simulink model "pcm"  (R2023b)
settings: Solver=VariableStepAuto  StartTime=0.0  StopTime=50  RelTol=1e-3
undefined symbols (not defined in the file): doppler
libraries: dspquant2 x2, dspfdesign x2, commchan3 x1
settings Model: Creator=HP  LastModifiedBy=HP

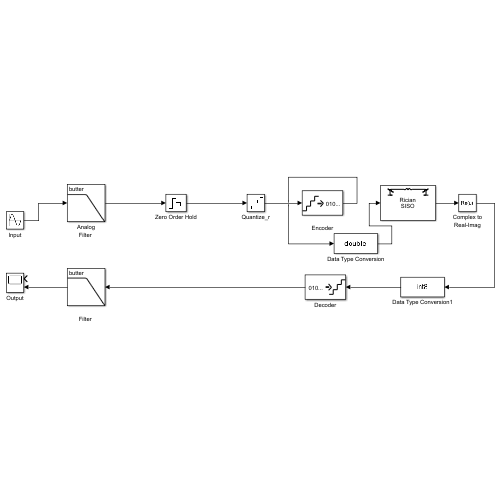
[thumbnail: Simulink's stored preview of the top-level diagram]
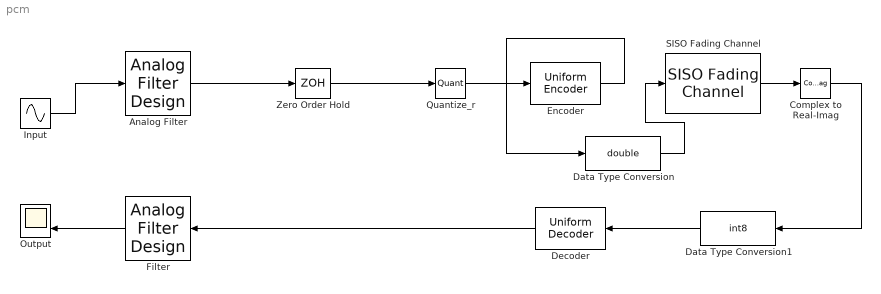
== system pcm ==
  " Encoder" : dspquant2/Uniform Encoder  peak=1  bits=3  otype=Unsigned integer
  " Filter " : dspfdesign/Analog Filter Design  method=Butterworth  filttype=Lowpass  N=8  Wlo=30  Whi=80  Rp=2  Rs=40
  "Analog Filter " : dspfdesign/Analog Filter Design  method=Butterworth  filttype=Lowpass  N=8  Wlo=30  Whi=80  Rp=2  Rs=40
  Complex to Real-Imag : ComplexToRealImag  Output=Real
  Data Type Conversion : DataTypeConversion  OutDataTypeStr=double  SaturateOnIntegerOverflow=off  RndMeth=Floor
  Data Type Conversion1 : DataTypeConversion  OutDataTypeStr=int8  SaturateOnIntegerOverflow=off  RndMeth=Floor
  Decoder : dspquant2/Uniform Decoder  peak=1  bits=8  overflowMode=Saturate  otype=Double
  Input : Sin  Amplitude=5  Frequency=5  SampleTime=0
  Output : Scope  NumInputPorts=2
  Quantize_r : Quantizer  QuantizationInterval=1
  SISO Fading Channel : commchan3/SISO Fading Channel  InheritSampleRate=on  SampleRate=1  PathDelays=0  AveragePathGains=0  NormalizePathGains=on  FadingDistribution=Rician  KFactor=3  DirectPathDopplerShift=0  DirectPathInitialPhase=0  MaximumDopplerShift=0  DopplerSpectrum=doppler('Jakes')  RandomStream=mt19937ar with seed  Seed=75  PathGainsOutputPort=off  ChannelFilterDelayOutputPort=off  SimulateUsing=Interpreted execution  Visualization=Impulse response  PathsForDopplerDisplay=1  SamplesToDisplay=25%
  Zero Order Hold : ZeroOrderHold  SampleTime=-1
  wires:
  Decoder/1 -> " Filter "/1
  Input/1 -> "Analog Filter "/1
  "Analog Filter "/1 -> Zero Order Hold/1
  Zero Order Hold/1 -> Quantize_r/1
  Quantize_r/1 -> " Encoder"/1
  SISO Fading Channel/1 -> Complex to Real-Imag/1
  Complex to Real-Imag/1 -> Data Type Conversion1/1
  " Encoder"/1 -> Data Type Conversion/1
  Data Type Conversion/1 -> SISO Fading Channel/1
  Data Type Conversion1/1 -> Decoder/1
  " Filter "/1 -> Output/2
